simulink model "psoPID"  (R2024a)
settings: Solver=VariableStepAuto  StartTime=0.0  StopTime=10.0  RelTol=1e-3
values from neighbouring files (symbols this model uses):
  Kd = particle(1, 1, 3)    [psoFitFunction.m]
  Ki = particle(1, 1, 2)    [psoFitFunction.m]
  Kp = particle(1, 1, 1)    [psoFitFunction.m]
settings Model: Creator=oying  LastModifiedBy=oying

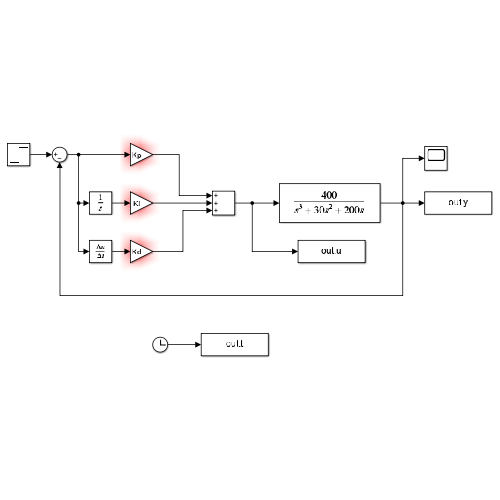
[thumbnail: Simulink's stored preview of the top-level diagram]
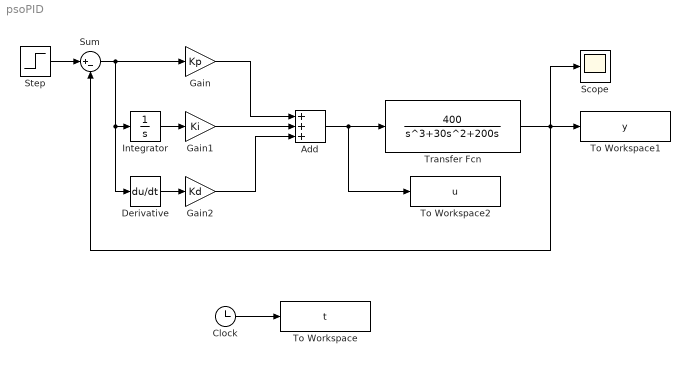
== system psoPID ==
  Add : Sum  Inputs=+++
  Clock : Clock
  Derivative : Derivative
  Gain : Gain  Gain=Kp
  Gain1 : Gain  Gain=Ki
  Gain2 : Gain  Gain=Kd
  Integrator : Integrator
  Scope : Scope
  Step : Step  SampleTime=0
  Sum : Sum  Inputs=|+-
  To Workspace : ToWorkspace  VariableName=t  SampleTime=-1
  To Workspace1 : ToWorkspace  VariableName=y  SampleTime=-1
  To Workspace2 : ToWorkspace  VariableName=u  SampleTime=-1
  Transfer Fcn : TransferFcn  Numerator=[400]  Denominator=[ 1 30 200 0]
  wires:
  Clock/1 -> To Workspace/1
  Step/1 -> Sum/1
  Sum/1 -> Integrator/1, Derivative/1, Gain/1
  Integrator/1 -> Gain1/1
  Derivative/1 -> Gain2/1
  Gain/1 -> Add/1
  Gain1/1 -> Add/2
  Gain2/1 -> Add/3
  Add/1 -> To Workspace2/1, Transfer Fcn/1
  Transfer Fcn/1 -> Scope/1, Sum/2, To Workspace1/1
